simulink model "Squelette_DSPBuilder"  (R2016a)
settings: Solver=VariableStepDiscrete  StartTime=0.0  StopTime=20e-6  RelTol=1e-3
InitFcn:
  | %% DSPBuilder Start
  | alt_dspbuilder_update_model(bdroot)
  | %% DSPBuilder End
libraries: allblocks_alteradspbuilder2 x20
settings Model: Creator=rhev2401  LastModifiedBy=dufd2703
settings DataIOCC: LimitDataPoints=on  SaveFormat=Array
settings DebuggingCC: SolverPrmCheckMsg=warning
settings HardwareCC: ProdBitPerPointer=32  ProdLargestAtomicFloat=None  ProdIntDivRoundTo=Undefined  ProdEndianess=Unspecified  ProdWordSize=32  ProdHWDeviceType=32-bit Generic
settings ModelReferenceCC: PropagateSignalLabelsOutOfModel=off
settings ConfigComp: CovModelRefEnable=Off  CovSFcnEnable=off

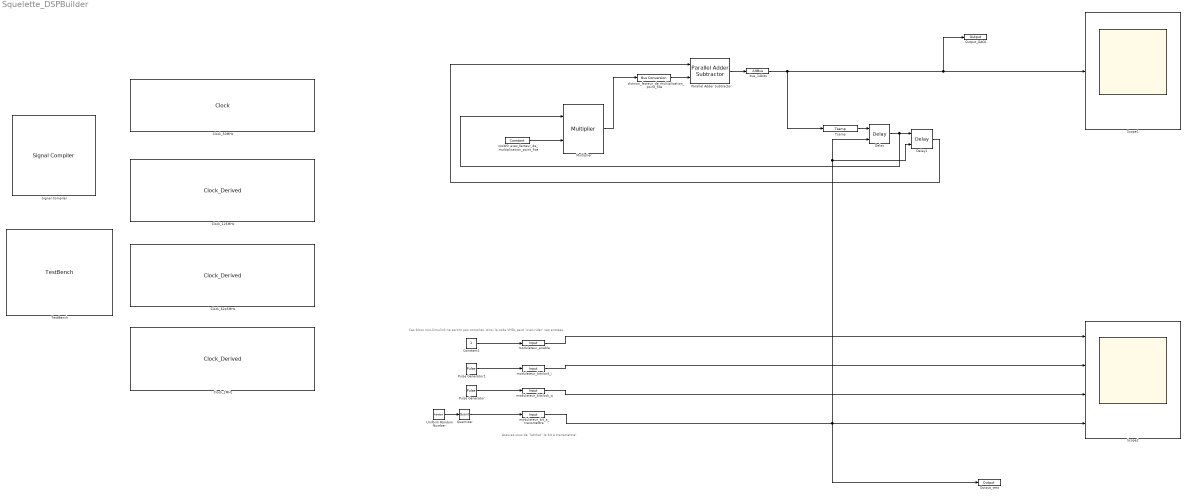
== system Squelette_DSPBuilder ==
  note: Ces blocs non-Simulink ne seront pas compilés. Ainsi le code VHDL peut "over-rider" ces entrées.
  note: Assurez-vous de "latcher" le bit à transmettre!
  Clock_125MHz : allblocks_alteradspbuilder2/Clock_Derived  ClockNumerator=2  ClockDenominator=5  ResetLatency=0  ResetRegisterCascadeDepth=0  SimulationStartCycle=5  PhaseOffset=0  Reset=aclr_125  ResetType=Active Low  Export=off
  Clock_2MHz : allblocks_alteradspbuilder2/Clock_Derived  ClockNumerator=25  ClockDenominator=1  ResetLatency=0  ResetRegisterCascadeDepth=0  SimulationStartCycle=5  PhaseOffset=0  Reset=aclr_2  ResetType=Active Low  Export=off
  Clock_50MHz : allblocks_alteradspbuilder2/Clock  ClockPeriod=20  ClockPeriodUnit=ns  SampleTime=20e-9  ResetLatency=0  ResetRegisterCascadeDepth=0  SimulationStartCycle=5  PhaseOffset=0  Reset=aclr  ResetType=Active Low  Export=off
  Clock_62p5MHz : allblocks_alteradspbuilder2/Clock_Derived  ClockNumerator=4  ClockDenominator=5  ResetLatency=0  ResetRegisterCascadeDepth=0  SimulationStartCycle=5  PhaseOffset=0  Reset=aclr_62p5  ResetType=Active Low  Export=off
  Constant1 : Constant
  Delay : allblocks_alteradspbuilder2/Delay  pipeline=1  pipeline_display=1  ClockPhase=1  use_ena=off  use_sclr=on  allowFloatingPointOverride=on  logOutputs=off  logFile=U:\projet-s6\DSP builder\2014-07-10-Squelette1\Squelette1\Squelette_Quartus\Squelette_DSPBuilder\tb_Squelette_DSPBuilder\Squelette%5FDSPBuilder_Delay.fixedpointlog  use_init=on  reset_value=y_n_1
  Delay1 : allblocks_alteradspbuilder2/Delay  pipeline=1  pipeline_display=1  ClockPhase=1  use_ena=off  use_sclr=on  allowFloatingPointOverride=on  logOutputs=off  logFile=U:\projet-s6\DSP builder\2014-07-10-Squelette1\Squelette1\Squelette_Quartus\Squelette_DSPBuilder\tb_Squelette_DSPBuilder\Squelette%5FDSPBuilder_Delay1.fixedpointlog  use_init=on  reset_value=y_n_2
  Multiplier : allblocks_alteradspbuilder2/Multiplier  BusType=Signed Integer  bwl=14  bwr=0  pipeline=0  pipeline_display=0  allowFloatingPointOverride=on  logOutputs=off  logFile=U:\projet-s6\DSP builder\2014-07-10-Squelette1\Squelette1\Squelette_Quartus\Squelette_DSPBuilder\tb_Squelette_DSPBuilder\Squelette%5FDSPBuilder_Multiplier.fixedpointlog  UseEqualInputWidth=off  bbwl=19  bbwr=0  FullResolution=on  OutputMsb=8  OutputLsb=0  OutputBwl=16  OutputBwr=16  UseDedicatedCircuitry=YES  use_ena=off  use_aclr=off
  Output_DAC0 : allblocks_alteradspbuilder2/Output  iofile=U:\projet-s6\DSP builder\2014-07-10-Squelette1\Squelette1\Squelette_Quartus\Squelette_DSPBuilder\tb_Squelette_DSPBuilder\Squelette%5FDSPBuilder_Output%5FDAC0.capture  BusType=Signed Integer  bwl=14  bwr=0  externalType=Inferred  PORTTYPE=Output  allowFloatingPointOverride=on  logOutputs=off
  Output_test : allblocks_alteradspbuilder2/Output  iofile=U:\projet-s6\DSP builder\2014-07-10-Squelette1\Squelette1\Squelette_Quartus\Squelette_DSPBuilder\tb_Squelette_DSPBuilder\Squelette%5FDSPBuilder_Output%5Ftest.capture  BusType=Single Bit  bwl=14  bwr=0  externalType=Inferred  PORTTYPE=Output  allowFloatingPointOverride=on  logOutputs=off
  Parallel Adder Subtractor : allblocks_alteradspbuilder2/Parallel Adder Subtractor  number_of_inputs=2  direction=-+  use_pipeline=off  pipeline_display=0  phase_selection=1  use_ena=off  use_aclr=off  allowFloatingPointOverride=on  logOutputs=off  logFile=U:\projet-s6\DSP builder\2014-07-10-Squelette1\Squelette1\Squelette_Quartus\Squelette_DSPBuilder\tb_Squelette_DSPBuilder\Squelette%5FDSPBuilder_Parallel+Adder+Subtractor.fixedpointlog
  Pulse Generator : DiscretePulseGenerator  PulseType=Time based  Period=1e-6  PulseWidth=0.8  PhaseDelay=5e-7
  Pulse Generator1 : DiscretePulseGenerator  PulseType=Time based  Period=1e-6  PulseWidth=0.8
  Quantizer : Quantizer  QuantizationInterval=1
  Scope1 : Scope
  Scope2 : Scope  NumInputPorts=4
  Signal Compiler : allblocks_alteradspbuilder2/Signal Compiler  DeviceFamily=Cyclone V  DeviceName=AUTO  DisableEarlyHDLGeneration=off  EnableSignalTap=off  SignalTapDepth=128  UseBoardBlock=off  StpUseDefaultClock=on  StpClock=Clock_50MHz  ExportDir=C:\altera\14.0\quartus\dsp_builder  MAX10_ProgrammingMode=Internal Flash (SDM) Single Boot
  TestBench : allblocks_alteradspbuilder2/TestBench  enable=on  advancedMode=on  modelSimGui=on  maxDisplayErrors=10  mismatchErrorLevel=Error  simdatafile=U:\projet-s6\DSP builder\2014-07-10-Squelette1\Squelette1\Squelette_Quartus\Squelette_DSPBuilder\tb_Squelette_DSPBuilder\Squelette_DSPBuilder.simdata.tcl
  Tsamp : allblocks_alteradspbuilder2/Tsamp  SpecifyClock=on  clock=Clock_125MHz
  Uniform Random Number : UniformRandomNumber  Minimum=0  Seed=2  SampleTime=5e-7
  bus_14bits : allblocks_alteradspbuilder2/AltBus  BusType=Signed Integer  bwl=14  bwr=0  saturate=off  floatingPointInput=on  floatingPointOutput=on  logOutputs=off  logFile=U:\projet-s6\DSP builder\2014-07-10-Squelette1\Squelette1\Squelette_Quartus\Squelette_DSPBuilder\tb_Squelette_DSPBuilder\Squelette%5FDSPBuilder_bus%5F14bits.fixedpointlog
  cosW0_avec_facteur_de_multiplication_point_fixe : allblocks_alteradspbuilder2/Constant  mask_cst=a1  BusType=Signed Integer  bwl=19  bwr=0  roundMode=Truncate  satMode=Wrap  SpecifyClock=off  allowFloatingPointOverride=on  logOutputs=off  logFile=U:\projet-s6\DSP builder\2014-07-10-Squelette1\Squelette1\Squelette_Quartus\Squelette_DSPBuilder\tb_Squelette_DSPBuilder\Squelette%5FDSPBuilder_cosW0%5Favec%5Ffacteur%5Fde%5Fmultiplication%5Fpoint%5Ffixe.fixedpointlog
  division_facteur_de_multiplication_point_fixe : allblocks_alteradspbuilder2/Bus Conversion  BusType=Signed Integer  ibwl=33  ibwr=1  bwl=14  bwr=1  bitToConnectToOutputLSB=16  round=off  saturate=off  pipeline_display=0
  modulateur_bit_a_transmettre : allblocks_alteradspbuilder2/Input  iofile=U:\projet-s6\DSP builder\2014-07-10-Squelette1\Squelette1\Squelette_Quartus\Squelette_DSPBuilder\tb_Squelette_DSPBuilder\Squelette%5FDSPBuilder_modulateur%5Fbit%5Fa%5Ftransmettre.salt  BusType=Single Bit  bwl=8  bwr=0  SpecifyClock=off  PORTTYPE=Input  externalType=Inferred  allowFloatingPointOverride=on  logOutputs=off
  modulateur_bitclock_i : allblocks_alteradspbuilder2/Input  iofile=U:\projet-s6\DSP builder\2014-07-10-Squelette1\Squelette1\Squelette_Quartus\Squelette_DSPBuilder\tb_Squelette_DSPBuilder\Squelette%5FDSPBuilder_modulateur%5Fbitclock%5Fi.salt  BusType=Single Bit  bwl=8  bwr=0  SpecifyClock=off  PORTTYPE=Input  externalType=Inferred  allowFloatingPointOverride=on  logOutputs=off
  modulateur_bitclock_q : allblocks_alteradspbuilder2/Input  iofile=U:\projet-s6\DSP builder\2014-07-10-Squelette1\Squelette1\Squelette_Quartus\Squelette_DSPBuilder\tb_Squelette_DSPBuilder\Squelette%5FDSPBuilder_modulateur%5Fbitclock%5Fq.salt  BusType=Single Bit  bwl=8  bwr=0  SpecifyClock=off  PORTTYPE=Input  externalType=Inferred  allowFloatingPointOverride=on  logOutputs=off
  modulateur_enable : allblocks_alteradspbuilder2/Input  iofile=U:\projet-s6\DSP builder\2014-07-10-Squelette1\Squelette1\Squelette_Quartus\Squelette_DSPBuilder\tb_Squelette_DSPBuilder\Squelette%5FDSPBuilder_modulateur%5Fenable.salt  BusType=Single Bit  bwl=8  bwr=0  SpecifyClock=off  PORTTYPE=Input  externalType=Inferred  allowFloatingPointOverride=on  logOutputs=off
  wires:
  Delay/1 -> Multiplier/1, Delay1/1
  cosW0_avec_facteur_de_multiplication_point_fixe/1 -> Multiplier/2
  Delay1/1 -> Parallel Adder Subtractor/1
  bus_14bits/1 -> Output_DAC0/1, Scope1/1, Tsamp/1
  Parallel Adder Subtractor/1 -> bus_14bits/1
  division_facteur_de_multiplication_point_fixe/1 -> Parallel Adder Subtractor/2
  Multiplier/1 -> division_facteur_de_multiplication_point_fixe/1
  Tsamp/1 -> Delay/1
  Constant1/1 -> modulateur_enable/1
  Pulse Generator1/1 -> modulateur_bitclock_i/1
  Pulse Generator/1 -> modulateur_bitclock_q/1
  Uniform Random Number/1 -> Quantizer/1
  Quantizer/1 -> modulateur_bit_a_transmettre/1
  modulateur_enable/1 -> Scope2/1
  modulateur_bitclock_i/1 -> Scope2/2
  modulateur_bitclock_q/1 -> Scope2/3
  modulateur_bit_a_transmettre/1 -> Output_test/1, Delay1/2, Delay/2, Scope2/4
